simulink model "pwm_half_output"  (R2021a)
settings: Solver=VariableStepAuto  StartTime=0.0  StopTime=0.2  RelTol=1e-4
libraries: spsIdealSwitchLib x6, spsSeriesRLCBranchLib x6, spsVoltageMeasurementLib x2, spsDCVoltageSourceLib x2, spsSawtoothGeneratorLib x2, spspowerguiLib x1
settings Model: Creator=Aluno  LastModifiedBy=Aluno
settings SolverCC: ZeroCrossAlgorithm=Adaptive
settings DebuggingCC: IgnoredZcDiagnostic=none

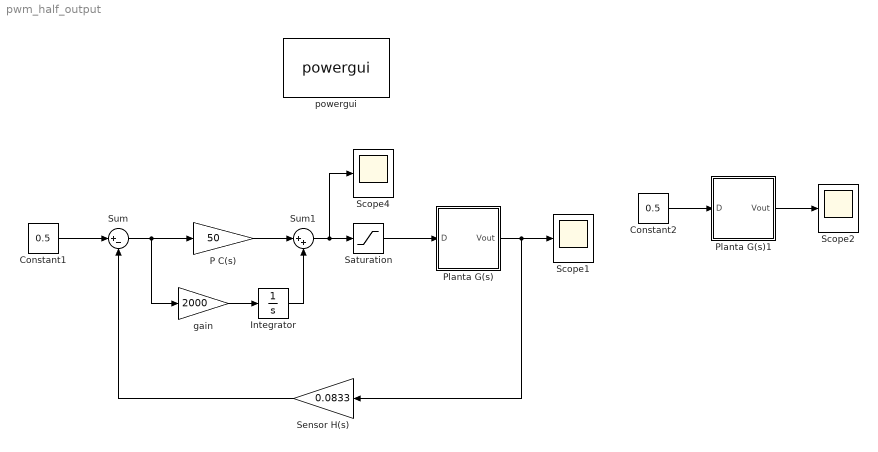
== system pwm_half_output ==
  Constant1 : Constant  Value=0.5
  Constant2 : Constant  Value=0.5
  Integrator : Integrator
  P C(s) : Gain  Gain=50
  Planta G(s) : Subsystem
  Planta G(s)1 : Subsystem
  Saturation : Saturate  UpperLimit=1  LowerLimit=0
  Scope1 : Scope
  Scope2 : Scope
  Scope4 : Scope
  Sensor H(s) : Gain  Gain=0.0833
  Sum : Sum  Inputs=|+-
  Sum1 : Sum  Inputs=|++
  gain : Gain  Gain=2000
  powergui : spspowerguiLib/powergui  Priority=1  SimulationMode=Continuous  SampleTime=50e-6  frequency=60  Iterations=50  frequencyindice=0  Pbase=100e6  ErrMax=1e-4  UnitsV=kV  UnitsW=MW  buscounter=0  FunctionMessages=off  echomessages=off  EnableUseOfTLC=off  CurrentSourceSwitches=off  DisableSnubberDevices=off  DisableRonSwitches=off  DisableVfSwitches=off  DisplayEquations=off  AutomaticDiscreteSolvers=off  SolverType=Tustin/Backward Euler (TBE)  Interpol=off  ExternalGateDelay=off  methode=off  Ts=100  x0status=blocks  SPID=on  SwTol=0  HookPort=off  NonlinearTolerance=1e-4  nMaxIteration=100  ContinueOnMaxIteration=off  RestoreLinks=warning  ResistiveCurrentMeasurement=off  Frange=[0:2:500]  Ylog=off  Xlog=on  ShowGrid=off  save=off  variable=ZData  structure=0  ZoomFFT=off  StartTime=0.0  cycles=1  DisplayStyle=1  fundamental=60  FreqAxis=off  MaxFrequency=1000  frequencyindicesteady=1  RmsSteady=1  display=off
  wires:
  Constant1/1 -> Sum/1
  Sum/1 -> gain/1, P C(s)/1
  Sensor H(s)/1 -> Sum/2
  Planta G(s)/1(Vout) -> Sensor H(s)/1, Scope1/1
  Constant2/1 -> Planta G(s)1/1(D)
  Planta G(s)1/1(Vout) -> Scope2/1
  Saturation/1 -> Planta G(s)/1(D)
  gain/1 -> Integrator/1
  P C(s)/1 -> Sum1/1
  Sum1/1 -> Scope4/1, Saturation/1
  Integrator/1 -> Sum1/2

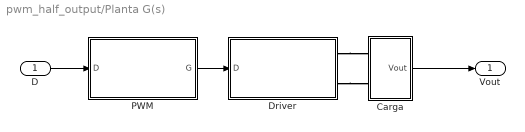
== system pwm_half_output/Planta G(s) ==
  D : Inport
  Carga : Subsystem
  Driver : Subsystem
  PWM : Subsystem
  Vout : Outport
  wires:
  PWM/1(G) -> Driver/1(D)
  D/1 -> PWM/1(D)
  Carga/1(Vout) -> Vout/1
  connections:
  Driver/RConn1 -- Carga/LConn1
  Driver/RConn2 -- Carga/LConn2

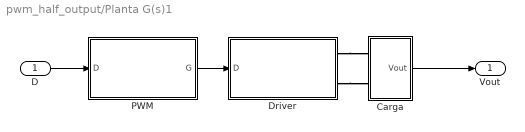
== system pwm_half_output/Planta G(s)1 ==
  D : Inport
  Carga : Subsystem
  Driver : Subsystem
  PWM : Subsystem
  Vout : Outport
  wires:
  Carga/1(Vout) -> Vout/1
  D/1 -> PWM/1(D)
  PWM/1(G) -> Driver/1(D)
  connections:
  Driver/RConn2 -- Carga/LConn2
  Driver/RConn1 -- Carga/LConn1

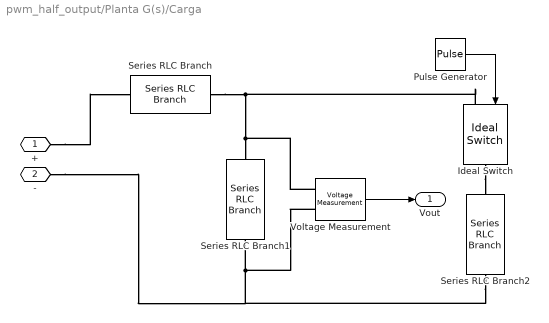
== system pwm_half_output/Planta G(s)/Carga ==
  Ideal Switch : spsIdealSwitchLib/Ideal Switch  Ron=0  Lon=0  IC=0  Rs=inf  Cs=inf  Measurements=off
  Pulse Generator : DiscretePulseGenerator  PulseType=Time based  Period=0.2  PulseWidth=10  PhaseDelay=0.1
  Series RLC Branch : spsSeriesRLCBranchLib/Series RLC Branch  LConnTagsString=__new0  RConnTagsString=__new0  BranchType=R  Resistance=1200  Inductance=1e-3  SetiL0=off  InitialCurrent=0  Capacitance=1e-6  Setx0=off  InitialVoltage=0  Measurements=None
  Series RLC Branch1 : spsSeriesRLCBranchLib/Series RLC Branch  LConnTagsString=__new0  RConnTagsString=__new0  BranchType=C  Resistance=1200  Inductance=1e-3  SetiL0=off  InitialCurrent=0  Capacitance=1e-6  Setx0=on  InitialVoltage=0  Measurements=None
  Series RLC Branch2 : spsSeriesRLCBranchLib/Series RLC Branch  LConnTagsString=__new0  RConnTagsString=__new0  BranchType=R  Resistance=2400  Inductance=1e-3  SetiL0=off  InitialCurrent=0  Capacitance=1e-6  Setx0=off  InitialVoltage=0  Measurements=None
  Voltage Measurement : spsVoltageMeasurementLib/Voltage Measurement  PhasorSimulation=off  OutputType=Complex  PSBequivalent=0
  + : PMIOPort  Side=Left
  - : PMIOPort  Port=2  Side=Left
  Vout : Outport
  wires:
  Voltage Measurement/1 -> Vout/1
  Pulse Generator/1 -> Ideal Switch/1
  connections:
  -/RConn1 -- Series RLC Branch2/LConn1 -- Voltage Measurement/LConn2 -- Series RLC Branch1/RConn1
  Series RLC Branch/LConn1 -- Ideal Switch/LConn1 -- Voltage Measurement/LConn1 -- Series RLC Branch1/LConn1
  Ideal Switch/RConn1 -- Series RLC Branch2/RConn1
  +/RConn1 -- Series RLC Branch/RConn1

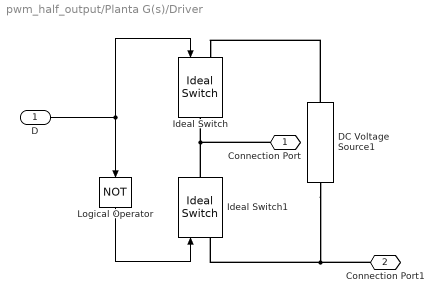
== system pwm_half_output/Planta G(s)/Driver ==
  D : Inport
  DC Voltage Source1 : spsDCVoltageSourceLib/DC Voltage Source  Amplitude=12  Measurements=None
  Ideal Switch : spsIdealSwitchLib/Ideal Switch  Ron=0  Lon=0  IC=0  Rs=inf  Cs=inf  Measurements=off
  Ideal Switch1 : spsIdealSwitchLib/Ideal Switch  Ron=0  Lon=0  IC=0  Rs=inf  Cs=inf  Measurements=off
  Logical Operator : Logic  Operator=NOT  AllPortsSameDT=off  OutDataTypeStr=boolean
  Connection Port : PMIOPort  Side=Right
  Connection Port1 : PMIOPort  Port=2  Side=Right
  wires:
  D/1 -> Ideal Switch/1, Logical Operator/1
  Logical Operator/1 -> Ideal Switch1/1
  connections:
  Ideal Switch1/RConn1 -- Connection Port/RConn1 -- Ideal Switch/RConn1
  Ideal Switch1/LConn1 -- Connection Port1/RConn1 -- DC Voltage Source1/LConn1
  DC Voltage Source1/RConn1 -- Ideal Switch/LConn1

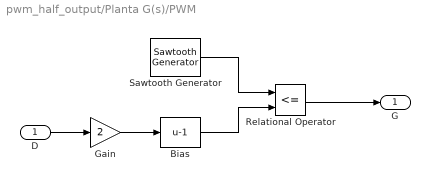
== system pwm_half_output/Planta G(s)/PWM ==
  D : Inport
  Bias : Bias  Bias=-1
  Gain : Gain  Gain=2
  Relational Operator : RelationalOperator  Operator=<=  OutDataTypeStr=boolean  RndMeth=Simplest
  Sawtooth Generator : spsSawtoothGeneratorLib/Sawtooth Generator  Freq=10000  Phase=180  Ts=0
  G : Outport
  wires:
  Sawtooth Generator/1 -> Relational Operator/1
  Relational Operator/1 -> G/1
  D/1 -> Gain/1
  Gain/1 -> Bias/1
  Bias/1 -> Relational Operator/2

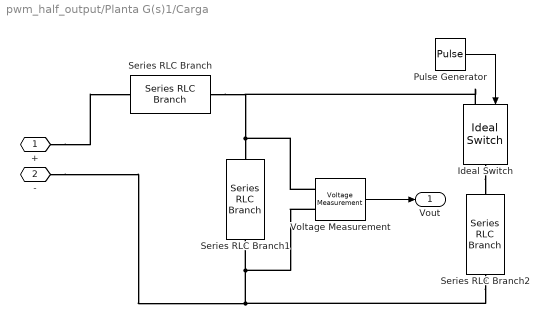
== system pwm_half_output/Planta G(s)1/Carga ==
  Ideal Switch : spsIdealSwitchLib/Ideal Switch  Ron=0  Lon=0  IC=0  Rs=inf  Cs=inf  Measurements=off
  Pulse Generator : DiscretePulseGenerator  PulseType=Time based  Period=0.2  PulseWidth=10  PhaseDelay=0.1
  Series RLC Branch : spsSeriesRLCBranchLib/Series RLC Branch  LConnTagsString=__new0  RConnTagsString=__new0  BranchType=R  Resistance=1200  Inductance=1e-3  SetiL0=off  InitialCurrent=0  Capacitance=1e-6  Setx0=off  InitialVoltage=0  Measurements=None
  Series RLC Branch1 : spsSeriesRLCBranchLib/Series RLC Branch  LConnTagsString=__new0  RConnTagsString=__new0  BranchType=C  Resistance=1200  Inductance=1e-3  SetiL0=off  InitialCurrent=0  Capacitance=1e-6  Setx0=on  InitialVoltage=0  Measurements=None
  Series RLC Branch2 : spsSeriesRLCBranchLib/Series RLC Branch  LConnTagsString=__new0  RConnTagsString=__new0  BranchType=R  Resistance=2400  Inductance=1e-3  SetiL0=off  InitialCurrent=0  Capacitance=1e-6  Setx0=off  InitialVoltage=0  Measurements=None
  Voltage Measurement : spsVoltageMeasurementLib/Voltage Measurement  PhasorSimulation=off  OutputType=Complex  PSBequivalent=0
  + : PMIOPort  Side=Left
  - : PMIOPort  Port=2  Side=Left
  Vout : Outport
  wires:
  Pulse Generator/1 -> Ideal Switch/1
  Voltage Measurement/1 -> Vout/1
  connections:
  +/RConn1 -- Series RLC Branch/RConn1
  Ideal Switch/RConn1 -- Series RLC Branch2/RConn1
  Voltage Measurement/LConn1 -- Series RLC Branch/LConn1 -- Ideal Switch/LConn1 -- Series RLC Branch1/LConn1
  -/RConn1 -- Series RLC Branch1/RConn1 -- Voltage Measurement/LConn2 -- Series RLC Branch2/LConn1

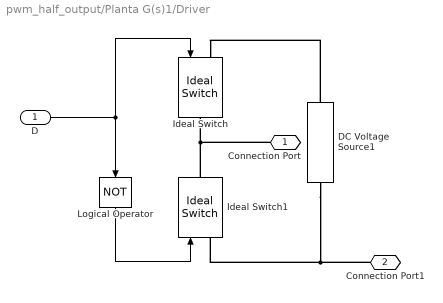
== system pwm_half_output/Planta G(s)1/Driver ==
  D : Inport
  DC Voltage Source1 : spsDCVoltageSourceLib/DC Voltage Source  Amplitude=12  Measurements=None
  Ideal Switch : spsIdealSwitchLib/Ideal Switch  Ron=0  Lon=0  IC=0  Rs=inf  Cs=inf  Measurements=off
  Ideal Switch1 : spsIdealSwitchLib/Ideal Switch  Ron=0  Lon=0  IC=0  Rs=inf  Cs=inf  Measurements=off
  Logical Operator : Logic  Operator=NOT  AllPortsSameDT=off  OutDataTypeStr=boolean
  Connection Port : PMIOPort  Side=Right
  Connection Port1 : PMIOPort  Port=2  Side=Right
  wires:
  Logical Operator/1 -> Ideal Switch1/1
  D/1 -> Logical Operator/1, Ideal Switch/1
  connections:
  DC Voltage Source1/RConn1 -- Ideal Switch/LConn1
  Connection Port1/RConn1 -- Ideal Switch1/LConn1 -- DC Voltage Source1/LConn1
  Connection Port/RConn1 -- Ideal Switch/RConn1 -- Ideal Switch1/RConn1

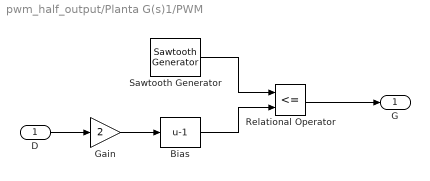
== system pwm_half_output/Planta G(s)1/PWM ==
  D : Inport
  Bias : Bias  Bias=-1
  Gain : Gain  Gain=2
  Relational Operator : RelationalOperator  Operator=<=  OutDataTypeStr=boolean  RndMeth=Simplest
  Sawtooth Generator : spsSawtoothGeneratorLib/Sawtooth Generator  Freq=10000  Phase=180  Ts=0
  G : Outport
  wires:
  Bias/1 -> Relational Operator/2
  Gain/1 -> Bias/1
  D/1 -> Gain/1
  Relational Operator/1 -> G/1
  Sawtooth Generator/1 -> Relational Operator/1
